simulink model "venkat"  (Simulink 6.6)
settings: Solver=ode45  StartTime=0.0  StopTime=0.01  RelTol=1e-3
libraries: powerlib x12, simulink x1
settings Model: Creator=Y9EE1238  LastModifiedBy=Y9EE1238

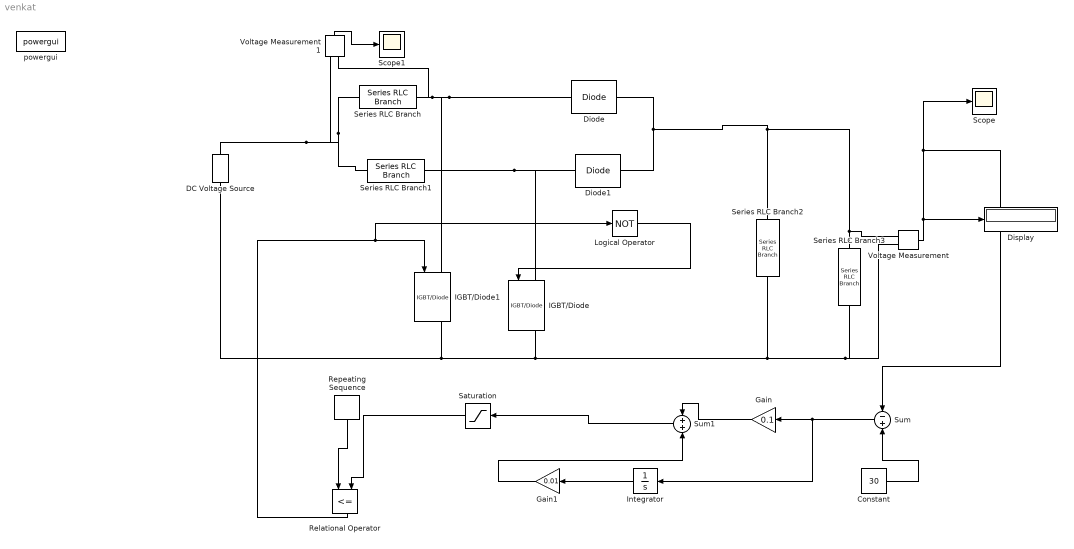
== system venkat ==
  Constant : Constant  Value=30
  DC Voltage Source : powerlib/Electrical Sources/DC Voltage Source  Orientation=up  DialogController=POWERSYS.PowerSysDialog  SystemSampleTime=-1  Amplitude=20  Measurements=None
  Diode : powerlib/Power Electronics/Diode  DialogController=POWERSYS.PowerSysDialog  SystemSampleTime=-1  Ron=0.001  Lon=0  Vf=0.01  IC=0  Rs=500  Cs=250e-9  Measurements=off
  Diode1 : powerlib/Power Electronics/Diode  DialogController=POWERSYS.PowerSysDialog  SystemSampleTime=-1  Ron=0.001  Lon=0  Vf=0.01  IC=0  Rs=500  Cs=250e-9  Measurements=off
  Display : Display
  Gain : Gain  Orientation=left  Gain=0.1
  Gain1 : Gain  Orientation=left  Gain=0.01
  IGBT/Diode : powerlib/Power Electronics/IGBT//Diode  Orientation=down  DialogController=POWERSYS.PowerSysDialog  SystemSampleTime=-1  Ron=1e-3  Rs=1e5  Cs=inf  Measurements=on
  IGBT/Diode1 : powerlib/Power Electronics/IGBT//Diode  Orientation=down  DialogController=POWERSYS.PowerSysDialog  SystemSampleTime=-1  Ron=1e-3  Rs=1e5  Cs=inf  Measurements=on
  Integrator : Integrator  Orientation=left
  Logical Operator : Logic  Operator=NOT  AllPortsSameDT=off  OutDataTypeMode=Boolean
  Relational Operator : RelationalOperator  Orientation=down  Operator=<=  LogicOutDataTypeMode=Boolean
  Repeating Sequence : simulink/Sources/Repeating Sequence  Orientation=down  SystemSampleTime=-1  rep_seq_t=[0 1/1000 1/1000]  rep_seq_y=[0 1 0]
  Saturation : Saturate  Orientation=left
  Scope : Scope
      settings: YMin=38.9  YMax=39.3
  Scope1 : Scope
      settings: TimeRange=6.063830196689768e-006  YMin=18.9888  YMax=20.9876
  Series RLC Branch : powerlib/Elements/Series RLC Branch  DialogController=POWERSYS.PowerSysDialog  PhysicalDomain=powersysdomain  SubClassName=unknown  LeftPortType=p1  RightPortType=p1  LConnTagsString=__new0  RConnTagsString=__new0  BranchType=L  Resistance=1  Inductance=[6.8e-3]  SetiL0=off  InitialCurrent=0  Capacitance=1e-6  Setx0=off  InitialVoltage=0  Measurements=None
  Series RLC Branch1 : powerlib/Elements/Series RLC Branch  DialogController=POWERSYS.PowerSysDialog  PhysicalDomain=powersysdomain  SubClassName=unknown  LeftPortType=p1  RightPortType=p1  LConnTagsString=__new0  RConnTagsString=__new0  BranchType=L  Resistance=1  Inductance=6.8e-3  SetiL0=off  InitialCurrent=0  Capacitance=1e-6  Setx0=off  InitialVoltage=0  Measurements=None
  Series RLC Branch2 : powerlib/Elements/Series RLC Branch  Orientation=down  DialogController=POWERSYS.PowerSysDialog  PhysicalDomain=powersysdomain  SubClassName=unknown  LeftPortType=p1  RightPortType=p1  LConnTagsString=__new0  RConnTagsString=__new0  BranchType=C  Resistance=1  Inductance=1e-3  SetiL0=off  InitialCurrent=0  Capacitance=750e-6  Setx0=off  InitialVoltage=0  Measurements=None
  Series RLC Branch3 : powerlib/Elements/Series RLC Branch  Orientation=down  DialogController=POWERSYS.PowerSysDialog  PhysicalDomain=powersysdomain  SubClassName=unknown  LeftPortType=p1  RightPortType=p1  LConnTagsString=__new0  RConnTagsString=__new0  BranchType=R  Resistance=16  Inductance=1e-3  SetiL0=off  InitialCurrent=0  Capacitance=1e-6  Setx0=off  InitialVoltage=0  Measurements=None
  Sum : Sum  Orientation=left  Inputs=-+
  Sum1 : Sum  Orientation=left
  Voltage Measurement : powerlib/Measurements/Voltage Measurement  DialogController=POWERSYS.PowerSysDialog  SystemSampleTime=-1  PhasorSimulation=off  OutputType=Complex  PSBequivalent=0
  Voltage Measurement1 : powerlib/Measurements/Voltage Measurement  Orientation=up  DialogController=POWERSYS.PowerSysDialog  SystemSampleTime=-1  PhasorSimulation=off  OutputType=Complex  PSBequivalent=0
  powergui : powerlib/powergui  SystemSampleTime=-1  SimulationMode=Discrete  SampleTime=50e-8  echomessages=off  RestoreLinks=warning  x0status=blocks  Frange=[0:2:500]  Ylog=off  Xlog=on  ShowGrid=off  save=off  variable=ZData  ZoomFFT=on  StartTime=0.0  cycles=1  DisplayStyle=1  fundamental=60  FreqAxis=off  MaxFrequency=1000  frequencyindice=0  frequencyindicesteady=1  RmsSteady=1  display=off  Ts=0  frequency=60  methode=off  HookPort=off  Interpol=off
  wires:
  Voltage Measurement/1 -> Display/1, Scope/1, Sum/1
  Voltage Measurement1/1 -> Scope1/1
  Constant/1 -> Sum/2
  Sum/1 -> Gain/1, Integrator/1
  Gain/1 -> Sum1/1
  Integrator/1 -> Gain1/1
  Gain1/1 -> Sum1/2
  Sum1/1 -> Saturation/1
  Repeating Sequence/1 -> Relational Operator/1
  Saturation/1 -> Relational Operator/2
  Relational Operator/1 -> IGBT/Diode1/1, Logical Operator/1
  Logical Operator/1 -> IGBT/Diode/1
  connections:
  DC Voltage Source/RConn1 -- Series RLC Branch1/LConn1 -- Series RLC Branch/LConn1 -- Voltage Measurement1/LConn1
  Series RLC Branch/RConn1 -- Diode/LConn1 -- IGBT/Diode1/LConn1 -- Voltage Measurement1/LConn2
  Series RLC Branch1/RConn1 -- Diode1/LConn1 -- IGBT/Diode/LConn1
  Diode/RConn1 -- Diode1/RConn1 -- Series RLC Branch2/LConn1 -- Series RLC Branch3/LConn1 -- Voltage Measurement/LConn1
  Series RLC Branch3/RConn1 -- Series RLC Branch2/RConn1 -- IGBT/Diode/RConn1 -- DC Voltage Source/LConn1 -- IGBT/Diode1/RConn1 -- Voltage Measurement/LConn2
